simulink model "fac_ut"  (Simulink 8.1)
settings: Solver=FixedStepDiscrete  StartTime=0.0  StopTime=Inf  FixedStep=0.005  RelTol=1e-3
libraries: fac x1
settings Model: Creator=xsellart  LastModifiedBy=AT015555
settings DataIOCC: SignalLoggingSaveFormat=Dataset
settings OptimizationCC: ExpressionDepthLimit=128
settings DebuggingCC: FcnCallInpInsideContextMsg=EnableAllAsError
settings GRTTargetCC: CombineOutputUpdateFcns=on  GRTInterface=off

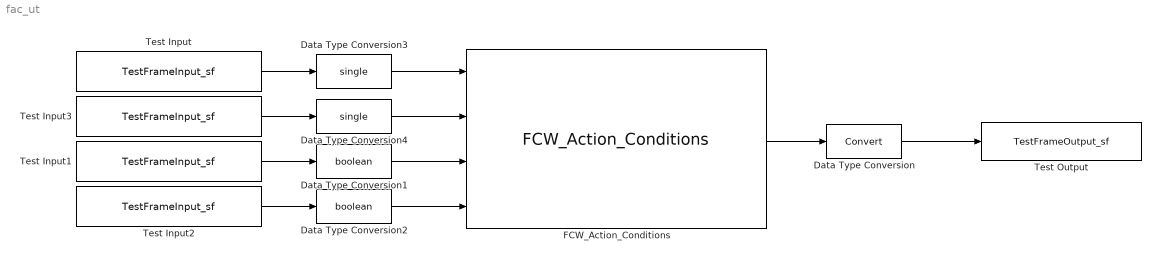
== system fac_ut ==
  Data Type Conversion : DataTypeConversion
  Data Type Conversion1 : DataTypeConversion  OutDataTypeStr=boolean
  Data Type Conversion2 : DataTypeConversion  OutDataTypeStr=boolean
  Data Type Conversion3 : DataTypeConversion  OutDataTypeStr=single
  Data Type Conversion4 : DataTypeConversion  OutDataTypeStr=single
  FCW_Action_Conditions : fac/FCW_Action_Conditions
  Test Input : S-Function  FunctionName=TestFrameInput_sf  Parameters=varname,sampletime  EnableBusSupport=off  mask(Test Input){varname=VJUD_FCWPointToWarn_m, sampletime=0.005}
      mask prompts: varname "Name:"; sampletime "Sample Time:"
      mask help: Outputs the value of a Test Input variable from an Excel spreadsheet when used with the runsiltest script. Otherwise outputs 0.
      mask Display: fprintf('Test Input:\n%s',varname);
  Test Input1 : S-Function  FunctionName=TestFrameInput_sf  Parameters=varname,sampletime  EnableBusSupport=off  mask(Test Input){varname=VIFO_FCWTargetVehAssigned_flg, sampletime=0.005}
      mask prompts: varname "Name:"; sampletime "Sample Time:"
      mask help: Outputs the value of a Test Input variable from an Excel spreadsheet when used with the runsiltest script. Otherwise outputs 0.
      mask Display: fprintf('Test Input:\n%s',varname);
  Test Input2 : S-Function  FunctionName=TestFrameInput_sf  Parameters=varname,sampletime  EnableBusSupport=off  mask(Test Input){varname=VAEB_AEBActingPrev_flg, sampletime=0.005}
      mask prompts: varname "Name:"; sampletime "Sample Time:"
      mask help: Outputs the value of a Test Input variable from an Excel spreadsheet when used with the runsiltest script. Otherwise outputs 0.
      mask Display: fprintf('Test Input:\n%s',varname);
  Test Input3 : S-Function  FunctionName=TestFrameInput_sf  Parameters=varname,sampletime  EnableBusSupport=off  mask(Test Input){varname=VIFO_FCWVehClearance_m, sampletime=0.005}
      mask prompts: varname "Name:"; sampletime "Sample Time:"
      mask help: Outputs the value of a Test Input variable from an Excel spreadsheet when used with the runsiltest script. Otherwise outputs 0.
      mask Display: fprintf('Test Input:\n%s',varname);
  Test Output : S-Function  FunctionName=TestFrameOutput_sf  Parameters=varname,sampletime  EnableBusSupport=off  mask(Test Output){varname=VJUD_FCWActionReq_flg, sampletime=-1}
      mask prompts: varname "Name:"; sampletime "Sample Time:"
      mask help: Samples the value of a Test Output variable from an Excel spreadsheet when used with the runsiltest script. Otherwise does nothing.
      mask Display: fprintf('Test Output:\n%s',varname);
  wires:
  FCW_Action_Conditions/1 -> Data Type Conversion/1
  Data Type Conversion/1 -> Test Output/1
  Test Input1/1 -> Data Type Conversion1/1
  Data Type Conversion1/1 -> FCW_Action_Conditions/3
  Test Input2/1 -> Data Type Conversion2/1
  Data Type Conversion2/1 -> FCW_Action_Conditions/4
  Test Input/1 -> Data Type Conversion3/1
  Data Type Conversion3/1 -> FCW_Action_Conditions/1
  Test Input3/1 -> Data Type Conversion4/1
  Data Type Conversion4/1 -> FCW_Action_Conditions/2
